simulink library "test_bench_lib"  (Simulink 9.2)
settings: Solver=VariableStepAuto  StartTime=0.0  StopTime=10.0  RelTol=1e-3
undefined symbols (not defined in the file or in its folder): p_max_bar
libraries: haley_test_bench_lib x1, dspfdesign x1
settings Model: Creator=habich  LastModifiedBy=entwicklungs-pc

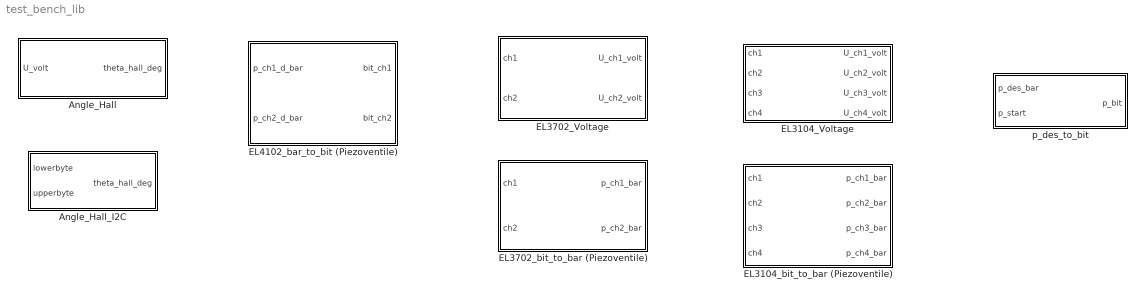
== system test_bench_lib ==
  Angle_Hall : MATLAB Function  TreatAsAtomicUnit=on
  Angle_Hall_I2C : Subsystem
  EL3104_Voltage : Subsystem
  EL3104_bit_to_bar (Piezoventile) : Subsystem
  EL3702_Voltage : Subsystem
  EL3702_bit_to_bar (Piezoventile) : Subsystem
  EL4102_bar_to_bit (Piezoventile) : MATLAB Function  TreatAsAtomicUnit=on
  p_des_to_bit : Subsystem

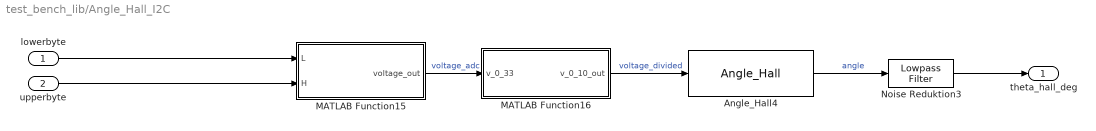
== system test_bench_lib/Angle_Hall_I2C ==
  lowerbyte : Inport
  upperbyte : Inport  Port=2
  Angle_Hall4 : haley_test_bench_lib/Angle_Hall  SystemSampleTime=-1
  MATLAB Function15 : MATLAB Function  TreatAsAtomicUnit=on
  MATLAB Function16 : MATLAB Function  TreatAsAtomicUnit=on
  Noise Reduktion3 : dspfdesign/Lowpass Filter  FilterType=FIR  DesignForMinimumOrder=on  FilterOrder=50  PassbandFrequency=0.1  StopbandFrequency=5  PassbandRipple=0.1  StopbandAttenuation=60  InheritSampleRate=off  SampleRate=1000  SimulateUsing=Interpreted execution  roundingMode=Floor  coeffsDataTypeStr=fixdt(1,16)
  theta_hall_deg : Outport
  wires:
  upperbyte/1 -> MATLAB Function15/2(H)
  Noise Reduktion3/1 -> theta_hall_deg/1
  Angle_Hall4/1 -> Noise Reduktion3/1  "angle"
  lowerbyte/1 -> MATLAB Function15/1(L)
  MATLAB Function16/1(v_0_10_out) -> Angle_Hall4/1  "voltage_divided"
  MATLAB Function15/1(voltage_out) -> MATLAB Function16/1(v_0_33)  "voltage_adc"

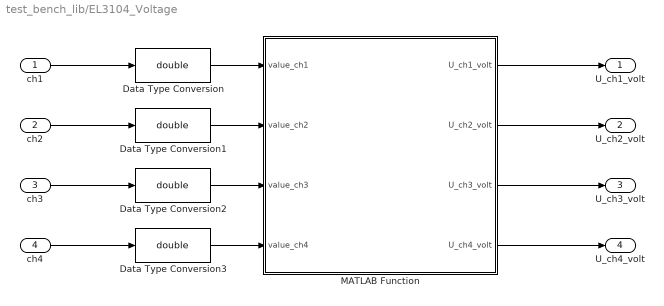
== system test_bench_lib/EL3104_Voltage ==
  ch1 : Inport
  ch2 : Inport  Port=2
  ch3 : Inport  Port=3
  ch4 : Inport  Port=4
  Data Type Conversion{,1..3} (4 alike) : DataTypeConversion  OutDataTypeStr=double
  MATLAB Function : MATLAB Function  TreatAsAtomicUnit=on
  U_ch1_volt : Outport
  U_ch2_volt : Outport  Port=2
  U_ch3_volt : Outport  Port=3
  U_ch4_volt : Outport  Port=4
  wires:
  ch1/1 -> Data Type Conversion/1
  ch2/1 -> Data Type Conversion1/1
  Data Type Conversion1/1 -> MATLAB Function/2(value_ch2)
  MATLAB Function/2(U_ch2_volt) -> U_ch2_volt/1
  Data Type Conversion/1 -> MATLAB Function/1(value_ch1)
  MATLAB Function/1(U_ch1_volt) -> U_ch1_volt/1
  Data Type Conversion2/1 -> MATLAB Function/3(value_ch3)
  ch3/1 -> Data Type Conversion2/1
  Data Type Conversion3/1 -> MATLAB Function/4(value_ch4)
  ch4/1 -> Data Type Conversion3/1
  MATLAB Function/3(U_ch3_volt) -> U_ch3_volt/1
  MATLAB Function/4(U_ch4_volt) -> U_ch4_volt/1

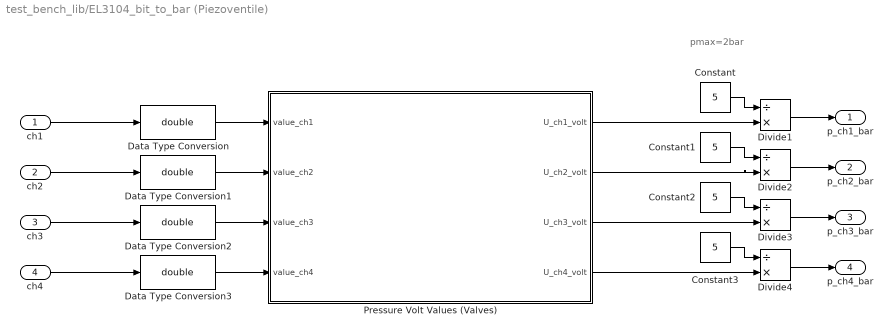
== system test_bench_lib/EL3104_bit_to_bar (Piezoventile) ==
  note: pmax=2bar
  ch1 : Inport
  ch2 : Inport  Port=2
  ch3 : Inport  Port=3
  ch4 : Inport  Port=4
  Constant{,1..3} (4 alike) : Constant  Value=5
  Data Type Conversion{,1..3} (4 alike) : DataTypeConversion  OutDataTypeStr=double
  Divide{1..4} (4 alike) : Product  Inputs=/*
  Pressure Volt Values (Valves) : MATLAB Function  TreatAsAtomicUnit=on
  p_ch1_bar : Outport
  p_ch2_bar : Outport  Port=2
  p_ch3_bar : Outport  Port=3
  p_ch4_bar : Outport  Port=4
  wires:
  Pressure Volt Values (Valves)/1(U_ch1_volt) -> Divide1/2
  Constant/1 -> Divide1/1
  Data Type Conversion1/1 -> Pressure Volt Values (Valves)/2(value_ch2)
  Divide1/1 -> p_ch1_bar/1
  ch2/1 -> Data Type Conversion1/1
  ch1/1 -> Data Type Conversion/1
  Data Type Conversion/1 -> Pressure Volt Values (Valves)/1(value_ch1)
  Data Type Conversion2/1 -> Pressure Volt Values (Valves)/3(value_ch3)
  ch3/1 -> Data Type Conversion2/1
  Data Type Conversion3/1 -> Pressure Volt Values (Valves)/4(value_ch4)
  ch4/1 -> Data Type Conversion3/1
  Pressure Volt Values (Valves)/2(U_ch2_volt) -> Divide2/2
  Divide2/1 -> p_ch2_bar/1
  Constant1/1 -> Divide2/1
  Pressure Volt Values (Valves)/3(U_ch3_volt) -> Divide3/2
  Divide3/1 -> p_ch3_bar/1
  Constant2/1 -> Divide3/1
  Pressure Volt Values (Valves)/4(U_ch4_volt) -> Divide4/2
  Divide4/1 -> p_ch4_bar/1
  Constant3/1 -> Divide4/1

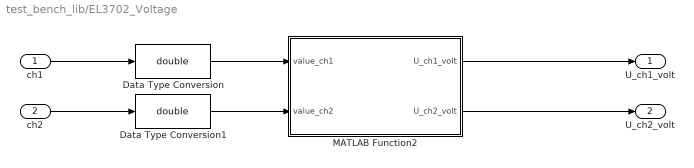
== system test_bench_lib/EL3702_Voltage ==
  "ch1 " : Inport
  ch2 : Inport  Port=2
  Data Type Conversion : DataTypeConversion  OutDataTypeStr=double
  Data Type Conversion1 : DataTypeConversion  OutDataTypeStr=double
  MATLAB Function2 : MATLAB Function  TreatAsAtomicUnit=on
  U_ch1_volt : Outport
  U_ch2_volt : Outport  Port=2
  wires:
  MATLAB Function2/1(U_ch1_volt) -> U_ch1_volt/1
  Data Type Conversion1/1 -> MATLAB Function2/2(value_ch2)
  ch2/1 -> Data Type Conversion1/1
  "ch1 "/1 -> Data Type Conversion/1
  Data Type Conversion/1 -> MATLAB Function2/1(value_ch1)
  MATLAB Function2/2(U_ch2_volt) -> U_ch2_volt/1

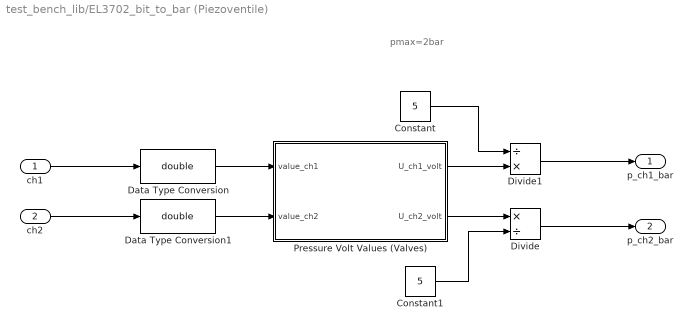
== system test_bench_lib/EL3702_bit_to_bar (Piezoventile) ==
  note: pmax=2bar
  "ch1 " : Inport
  ch2 : Inport  Port=2
  Constant : Constant  Value=5
  Constant1 : Constant  Value=5
  Data Type Conversion : DataTypeConversion  OutDataTypeStr=double
  Data Type Conversion1 : DataTypeConversion  OutDataTypeStr=double
  Divide : Product  Inputs=*/
  Divide1 : Product  Inputs=/*
  Pressure Volt Values (Valves) : MATLAB Function  TreatAsAtomicUnit=on
  p_ch1_bar : Outport
  p_ch2_bar : Outport  Port=2
  wires:
  "ch1 "/1 -> Data Type Conversion/1
  Pressure Volt Values (Valves)/2(U_ch2_volt) -> Divide/1
  ch2/1 -> Data Type Conversion1/1
  Pressure Volt Values (Valves)/1(U_ch1_volt) -> Divide1/2
  Constant/1 -> Divide1/1
  Divide1/1 -> p_ch1_bar/1
  Divide/1 -> p_ch2_bar/1
  Constant1/1 -> Divide/2
  Data Type Conversion/1 -> Pressure Volt Values (Valves)/1(value_ch1)
  Data Type Conversion1/1 -> Pressure Volt Values (Valves)/2(value_ch2)

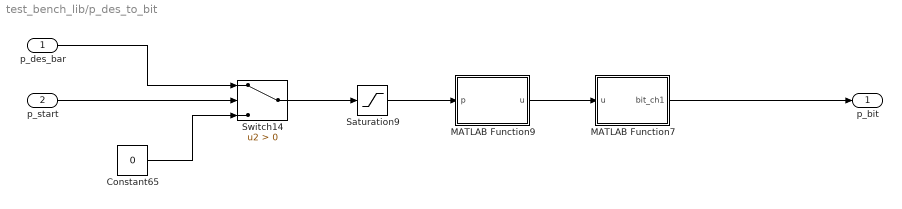
== system test_bench_lib/p_des_to_bit ==
  p_des_bar : Inport
  p_start : Inport  Port=2
  Constant65 : Constant  Value=0  SampleTime=1e-3
  MATLAB Function7 : MATLAB Function  TreatAsAtomicUnit=on
  MATLAB Function9 : MATLAB Function  TreatAsAtomicUnit=on
  Saturation9 : Saturate  UpperLimit=p_max_bar  LowerLimit=0
  Switch14 : Switch  Criteria=u2 > Threshold
  p_bit : Outport
  wires:
  Switch14/1 -> Saturation9/1
  Constant65/1 -> Switch14/3
  Saturation9/1 -> MATLAB Function9/1(p)
  p_des_bar/1 -> Switch14/1
  MATLAB Function7/1(bit_ch1) -> p_bit/1
  MATLAB Function9/1(u) -> MATLAB Function7/1(u)
  p_start/1 -> Switch14/2

== matlab function Angle_Hall ==
  data: U_volt input double; theta_hall_deg output double
function theta_hall_deg = fcn(U_volt)
theta_hall_deg= (U_volt*(1/9.99))*360

== matlab function EL3702_Voltage/MATLAB Function2 ==
  data: U_ch1_volt output double; value_ch1 input double; U_ch2_volt output double; value_ch2 input double
function [U_ch1_volt,U_ch2_volt] = Beckhoff_to_Voltage(value_ch1,value_ch2)
%Beckhoff EL3702 +-10V Analog Input 16 Bit
U_ch1_volt=10/32767*value_ch1;
U_ch2_volt=10/32767*value_ch2;

== matlab function EL4102_bar_to_bit (Piezoventile) ==
  data: p_ch1_d_bar input double; bit_ch1 output double; p_ch2_d_bar input double; bit_ch2 output double
function [bit_ch1,bit_ch2]= bar_to_bit(p_ch1_d_bar,p_ch2_d_bar)

Volt_1 = p_ch1_d_bar*5; %bar to Volt
Volt_2 = p_ch2_d_bar*5;

bit_ch1=Volt_1/10*32767; %to bit
bit_ch2=Volt_2/10*32767;

== matlab function EL3104_bit_to_bar (Piezoventile)/Pressure Volt Values (Valves) ==
  data: value_ch1 input double; U_ch1_volt output double; value_ch2 input double; value_ch3 input double; value_ch4 input double; U_ch2_volt output double; U_ch3_volt output double; U_ch4_volt output double
function [U_ch1_volt,U_ch2_volt,U_ch3_volt,U_ch4_volt] = Beckhoff_to_Voltage(value_ch1,value_ch2,value_ch3,value_ch4)
%Beckhoff EL3104 +-10V Analog Input 16 Bit
U_ch1_volt=10/32767*value_ch1;
U_ch2_volt=10/32767*value_ch2;
U_ch3_volt=10/32767*value_ch3;
U_ch4_volt=10/32767*value_ch4;

== matlab function EL3702_bit_to_bar (Piezoventile)/Pressure Volt Values (Valves) ==
  data: U_ch1_volt output double; value_ch1 input double; U_ch2_volt output double; value_ch2 input double
function [U_ch1_volt,U_ch2_volt] = Beckhoff_to_Voltage(value_ch1,value_ch2)
%Beckhoff EL3702 +-10V Analog Input 16 Bit
U_ch1_volt=10/32767*value_ch1;
U_ch2_volt=10/32767*value_ch2;

== matlab function EL3104_Voltage/MATLAB Function ==
  data: value_ch1 input double; U_ch1_volt output double; value_ch2 input double; U_ch2_volt output double; value_ch3 input double; value_ch4 input double; U_ch3_volt output double; U_ch4_volt output double
function [U_ch1_volt,U_ch2_volt,U_ch3_volt,U_ch4_volt] = Beckhoff_to_Voltage3104(value_ch1,value_ch2,value_ch3,value_ch4)
%Beckhoff EL3104 +-10V Analog Input 16 Bit
U_ch1_volt=10/32767*value_ch1;
U_ch2_volt=10/32767*value_ch2;
U_ch3_volt=10/32767*value_ch3;
U_ch4_volt=10/32767*value_ch4;

== matlab function p_des_to_bit/MATLAB Function7 ==
  data: u input double; bit_ch1 output double
function bit_ch1 = fcn(u)
bit_ch1=u/10*32768; %10V in 16 Bit signed Int

== matlab function p_des_to_bit/MATLAB Function9 ==
  data: p input double; u output double
function u = fcn(p)
    u = 0;
    if p<=2 %p_max = 2bar
        u= p*5; %bar to Volt
    end
end

== matlab function Angle_Hall_I2C/MATLAB Function15 ==
  data: L input uint8 size=1; H input uint8 size=1; voltage_out output double size=1
function voltage_out = concat_bitwise(L,H)                      
bit_word = [L,H];
int16_out = typecast(bit_word,'int16');                         %Low und High byte to 16 bit
voltage_out = (double(3.3)/double(4096))*double(int16_out);     %To Volt

== matlab function Angle_Hall_I2C/MATLAB Function16 ==
  data: v_0_33 input double; v_0_10_out output double
function v_0_10_out = map_voltage(v_0_33)
%reconstruct output voltage after voltage divider
v_0_10_out = v_0_33*(6800+3300)/3300; %divider: V_0_33 = V_0_10*R_2/(R_1+R_2). R1 = 6.8kOhm, R2=3.3kOhm
